simulink model "sistema"  (R2024a)
settings: Solver=VariableStepAuto  StartTime=0.0  StopTime=10.0  RelTol=1e-3
libraries: slpidlib x1
settings Model: Creator=user  LastModifiedBy=Elias
settings DebuggingCC: UnconnectedInputMsg=warning  UnconnectedOutputMsg=warning  UnconnectedLineMsg=warning
settings ModelReferenceCC: EnableRefExpFcnMdlSchedulingChecks=on
settings RTWCC: GPUComputeCapability=3.5  DLArmComputeVersion=19.05

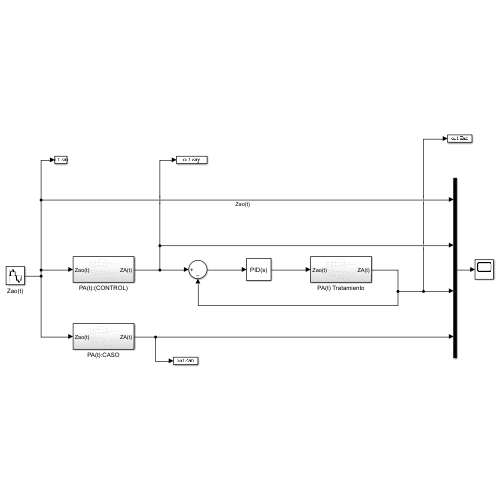
[thumbnail: Simulink's stored preview of the top-level diagram]
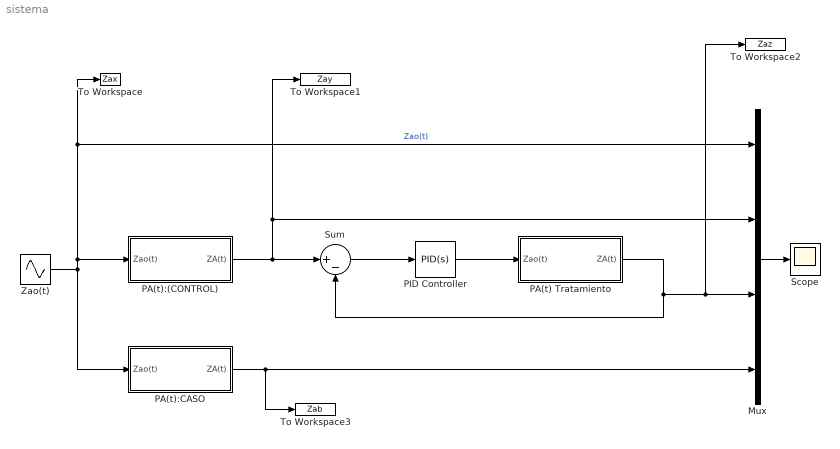
== system sistema ==
  Mux : Mux
  PA(t) Tratamiento : Subsystem
  PA(t):(CONTROL) : Subsystem
  PA(t):CASO : Subsystem
  PID Controller : slpidlib/PID Controller  Controller=PID  Form=Parallel  TimeDomain=Continuous-time  UseExternalTs=off  SampleTime=-1  IntegratorMethod=Forward Euler  FilterMethod=Forward Euler  ControllerParametersSource=internal  P=7504.31283990786  I=40028.7836532803  UseKiTs=off  D=312.586659285931  UseExternalDerivativeSource=off  N=104491.555602633  UseFilter=on  TunerSelectOption=Transfer Function Based (PID Tuner App)  InitialConditionSource=internal  InitialConditionForIntegrator=0  InitialConditionForFilter=0  DifferentiatorICPrevScaledInput=0  ExternalReset=none  TrackingMode=off  Kt=1  LimitOutput=off  SatLimitsSource=internal  UpperSaturationLimit=inf  LowerSaturationLimit=-inf  LinearizeAsGain=on  AntiWindupMode=none  Kb=1  LimitIntegrator=off  UpperIntegratorSaturationLimit=inf  LowerIntegratorSaturationLimit=-inf  POutMin=[]  POutMax=[]  IOutMin=[]  IOutMax=[]  DOutMin=[]  DOutMax=[]  NOutMin=[]  NOutMax=[]  SumOutMin=[]  SumOutMax=[]  SaturationOutMin=[]  SaturationOutMax=[]  PParamMin=[]  PParamMax=[]  IParamMin=[]  IParamMax=[]  DParamMin=[]  DParamMax=[]  NParamMin=[]  NParamMax=[]  KbParamMin=[]  KbParamMax=[]  KtParamMin=[]  KtParamMax=[]  KbOutMin=[]  KbOutMax=[]  KtOutMin=[]  KtOutMax=[]  IntegratorOutMin=[]  IntegratorOutMax=[]  FilterOutMin=[]  FilterOutMax=[]  SumI1OutMin=[]  SumI1OutMax=[]  SumI2OutMin=[]  SumI2OutMax=[]  SumI3OutMin=[]  SumI3OutMax=[]  SumI4OutMin=[]  SumI4OutMax=[]  SumDOutMin=[]  SumDOutMax=[]  DifferentiatorOutMin=[]  DifferentiatorOutMax=[]  FilterDiffOutCoefMin=[]  FilterDiffOutCoefMax=[]  ReciprocalOutMin=[]  ReciprocalOutMax=[]  SumDenOutMin=[]  SumDenOutMax=[]  SumNumOutMin=[]  SumNumOutMax=[]  DivideOutMin=[]  DivideOutMax=[]  UdiffTsProdOutMin=[]  UdiffTsProdOutMax=[]  NTsProdOutMin=[]  NTsProdOutMax=[]  UintegralTsProdOutMin=[]  UintegralTsProdOutMax=[]  UngainTsProdOutMin=[]  UngainTsProdOutMax=[]  ClampingZeroOutDataTypeStr=Inherit: Inherit via back propagation  ClampingZeroOutMin=[]  ClampingZeroOutMax=[]  FilterDenConstantOutDataTypeStr=Inherit: Inherit via back propagation  FilterDenConstantOutMin=[]  FilterDenConstantOutMax=[]  PCopyOutDataTypeStr=Inherit: Inherit via back propagation  PCopyOutMin=[]  PCopyOutMax=[]  NCopyOutDataTypeStr=Inherit: Inherit via back propagation  NCopyOutMin=[]  NCopyOutMax=[]  IntegratorContinuousStateAttributes=''  IntegratorStateMustResolveToSignalObject=off  IntegratorRTWStateStorageClass=Auto  FilterContinuousStateAttributes=''  FilterStateMustResolveToSignalObject=off  FilterRTWStateStorageClass=Auto  ParallelPVariant=InternalParameters  IdealPVariant=Disabled  IVariant=InternalParameters  DVariant=InternalParameters  IntegratorVariant=Continuous  SatVariant=Disabled  AWVariant=Passthrough  PCopyVariant=Disabled  TRVariant=Disabled  FdbkBlocksVariant=Forward  IdealPFdbkVariant=Disabled  SatFdbkVariant=Disabled  DerivativeFilterVariant=ContFilter  NVariant=InternalParameters  NCopyVariant=Disabled  FilterICVariant=InternalICsFilter  IntegratorICVariant=InternalICs  ExternalResetVariant=Disabled  TRSumVariant=Passthrough  SumFdbkVariant=Disabled  SumVariant=Sum_PID  TsampFilterVariant=InternalTs  TsampNgainVariant=Passthrough  TsampIntegralVariant=Disabled_SignalSpec  ExternalSaturationOutDataTypeStr=Inherit: Same as second input  DerivativeSourceVariant=ErrorSignal
  Scope : Scope
  Sum : Sum  Inputs=|+-
  To Workspace : ToWorkspace  VariableName=Zax  SampleTime=-1
      settings: Save2DSignal=2-D array (concatenate along first dimension)
  To Workspace1 : ToWorkspace  VariableName=Zay  SampleTime=-1
      settings: Save2DSignal=2-D array (concatenate along first dimension)
  To Workspace2 : ToWorkspace  VariableName=Zaz  SampleTime=-1
      settings: Save2DSignal=2-D array (concatenate along first dimension)
  To Workspace3 : ToWorkspace  VariableName=Zab  SampleTime=-1
      settings: Save2DSignal=2-D array (concatenate along first dimension)
  Zao(t) : Sin  Frequency=3.1416  SampleTime=0.001
  wires:
  Sum/1 -> PID Controller/1
  Mux/1 -> Scope/1
  PA(t) Tratamiento/1(ZA(t)) -> Sum/2, To Workspace2/1, Mux/3
  PA(t):CASO/1(ZA(t)) -> To Workspace3/1, Mux/4
  PA(t):(CONTROL)/1(ZA(t)) -> Sum/1, Mux/2, To Workspace1/1
  PID Controller/1 -> PA(t) Tratamiento/1(Zao(t))
  Zao(t)/1 -> To Workspace/1, Mux/1, PA(t):(CONTROL)/1(Zao(t)), PA(t):CASO/1(Zao(t))  "Zao(t)"

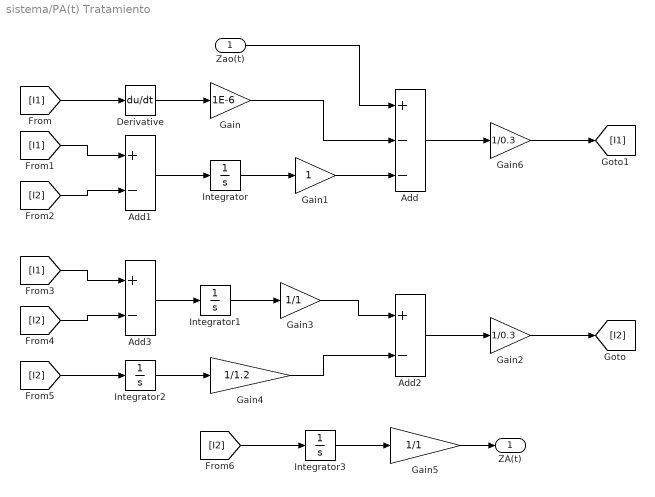
== system sistema/PA(t) Tratamiento ==
  Zao(t) : Inport
  Add : Sum  Inputs=+--
  Add1 : Sum  Inputs=+-
  Add2 : Sum  Inputs=+-
  Add3 : Sum  Inputs=+-
  Derivative : Derivative
  Gain : Gain  Gain=1E-6
  Gain1 : Gain
  Gain2 : Gain  Gain=1/0.3
  Gain3 : Gain  Gain=1/1
  Gain4 : Gain  Gain=1/1.2
  Gain5 : Gain  Gain=1/1
  Gain6 : Gain  Gain=1/0.3
  Integrator{,1..3} (4 alike) : Integrator
  ZA(t) : Outport
  wires:
  [I1] -> Derivative/1
  Derivative/1 -> Gain/1
  [I1] -> Add1/1
  [I2] -> Add1/2
  Add2/1 -> Gain2/1
  Gain2/1 -> [I2]
  [I2] -> Add3/2
  [I1] -> Add3/1
  Gain3/1 -> Add2/1
  Add1/1 -> Integrator/1
  Integrator/1 -> Gain1/1
  Add3/1 -> Integrator1/1
  Integrator1/1 -> Gain3/1
  [I2] -> Integrator2/1
  Integrator2/1 -> Gain4/1
  Gain4/1 -> Add2/2
  [I2] -> Integrator3/1
  Integrator3/1 -> Gain5/1
  Gain5/1 -> ZA(t)/1
  Gain1/1 -> Add/3
  Gain/1 -> Add/2
  Zao(t)/1 -> Add/1
  Add/1 -> Gain6/1
  Gain6/1 -> [I1]

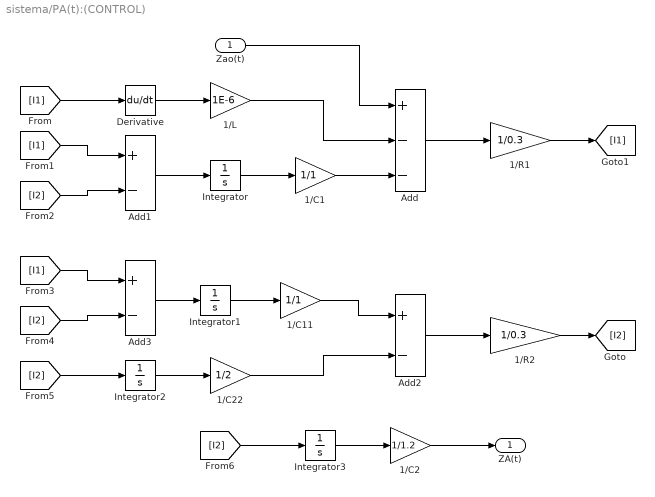
== system sistema/PA(t):(CONTROL) ==
  Zao(t) : Inport
  1/C1 : Gain  Gain=1/1
  1/C11 : Gain  Gain=1/1
  1/C2 : Gain  Gain=1/1.2
  1/C22 : Gain  Gain=1/2
  1/L : Gain  Gain=1E-6
  1/R1 : Gain  Gain=1/0.3
  1/R2 : Gain  Gain=1/0.3
  Add : Sum  Inputs=+--
  Add1 : Sum  Inputs=+-
  Add2 : Sum  Inputs=+-
  Add3 : Sum  Inputs=+-
  Derivative : Derivative
  Integrator{,1..3} (4 alike) : Integrator
  ZA(t) : Outport
  wires:
  [I1] -> Derivative/1
  Derivative/1 -> 1/L/1
  [I1] -> Add1/1
  [I2] -> Add1/2
  Add2/1 -> 1/R2/1
  1/R2/1 -> [I2]
  [I2] -> Add3/2
  [I1] -> Add3/1
  1/C11/1 -> Add2/1
  Add1/1 -> Integrator/1
  Integrator/1 -> 1/C1/1
  Add3/1 -> Integrator1/1
  Integrator1/1 -> 1/C11/1
  [I2] -> Integrator2/1
  Integrator2/1 -> 1/C22/1
  1/C22/1 -> Add2/2
  [I2] -> Integrator3/1
  Integrator3/1 -> 1/C2/1
  1/C2/1 -> ZA(t)/1
  1/C1/1 -> Add/3
  1/L/1 -> Add/2
  Zao(t)/1 -> Add/1
  Add/1 -> 1/R1/1
  1/R1/1 -> [I1]

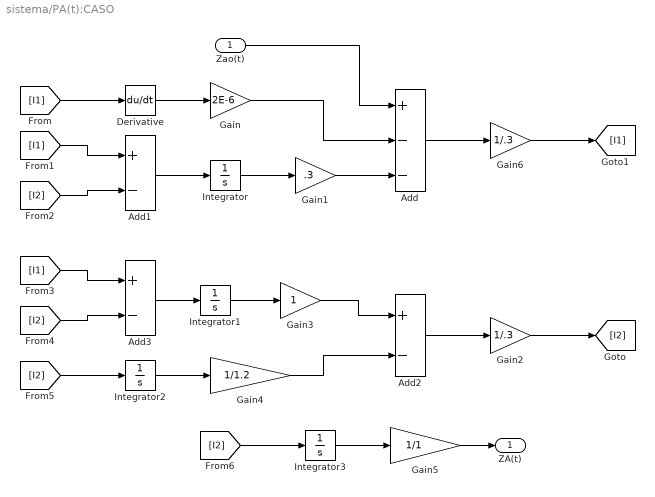
== system sistema/PA(t):CASO ==
  Zao(t) : Inport
  Add : Sum  Inputs=+--
  Add1 : Sum  Inputs=+-
  Add2 : Sum  Inputs=+-
  Add3 : Sum  Inputs=+-
  Derivative : Derivative
  Gain : Gain  Gain=2E-6
  Gain1 : Gain  Gain=.3
  Gain2 : Gain  Gain=1/.3
  Gain3 : Gain
  Gain4 : Gain  Gain=1/1.2
  Gain5 : Gain  Gain=1/1
  Gain6 : Gain  Gain=1/.3
  Integrator{,1..3} (4 alike) : Integrator
  ZA(t) : Outport
  wires:
  [I1] -> Derivative/1
  Derivative/1 -> Gain/1
  [I1] -> Add1/1
  [I2] -> Add1/2
  Add2/1 -> Gain2/1
  Gain2/1 -> [I2]
  [I2] -> Add3/2
  [I1] -> Add3/1
  Gain3/1 -> Add2/1
  Add1/1 -> Integrator/1
  Integrator/1 -> Gain1/1
  Add3/1 -> Integrator1/1
  Integrator1/1 -> Gain3/1
  [I2] -> Integrator2/1
  Integrator2/1 -> Gain4/1
  Gain4/1 -> Add2/2
  [I2] -> Integrator3/1
  Integrator3/1 -> Gain5/1
  Gain5/1 -> ZA(t)/1
  Gain1/1 -> Add/3
  Gain/1 -> Add/2
  Zao(t)/1 -> Add/1
  Add/1 -> Gain6/1
  Gain6/1 -> [I1]
